simulink model "M10B39"  (R2016b)
settings: Solver=ode23tb  StartTime=0.0  StopTime=20  FixedStep=0.001  MaxStep=0.01  RelTol=1e-3  EnableMultiTasking=on
InitFcn:
  | initAll
values from neighbouring files (symbols this model uses):
  SgridB = 100    [initAll.m]
  wB = 2*pi*fB    (= 314.159265359)    [initAll.m]
  YY_load = full(YY)    [powerflowcaculate.m]
undefined symbols (not defined in the file): Geninit
libraries: powerlib_meascontrol x10, simulink x1
(part 1 of 3)
settings Model: Creator=m  LastModifiedBy=LinSiQi
settings DataIOCC: LimitDataPoints=on  SaveFormat=Array  SignalLoggingSaveFormat=ModelDataLogs  SignalLoggingName=sigsOut
settings OptimizationCC: ExpressionDepthLimit=2147483647  LifeSpan=inf
settings DebuggingCC: SaveWithParameterizedLinksMsg=none  UnderspecifiedInitializationDetection=Classic  MergeDetectMultiDrivingBlocksExec=none  SignalResolutionControl=TryResolveAllWithWarning  MultiTaskDSMMsg=warning  MultiTaskCondExecSysMsg=none  FcnCallInpInsideContextMsg=warning  StateNameClashWarn=warning  SFUnexpectedBacktrackingDiag=warning  SFNoUnconditionalDefaultTransitionDiag=warning  SFExecutionAtInitializationDiag=none
settings HardwareCC: ProdBitPerPointer=32  ProdBitPerSizeT=32  ProdBitPerPtrDiffT=32  ProdLargestAtomicFloat=None  ProdIntDivRoundTo=Undefined  ProdEndianess=Unspecified  ProdWordSize=32  ProdHWDeviceType=32-bit Generic  TargetUnknown=on
settings ModelReferenceCC: PropagateSignalLabelsOutOfModel=off
settings GRTTargetCC: TargetLangStandard=C89/C90 (ANSI)  CombineOutputUpdateFcns=off  GRTInterface=on
settings ConfigComp: CovMetricSettings=dw  CovSaveCumulativeToWorkspaceVar=on  CovSaveSingleToWorkspaceVar=on  CovExternalEMLEnable=off  CovSFcnEnable=off

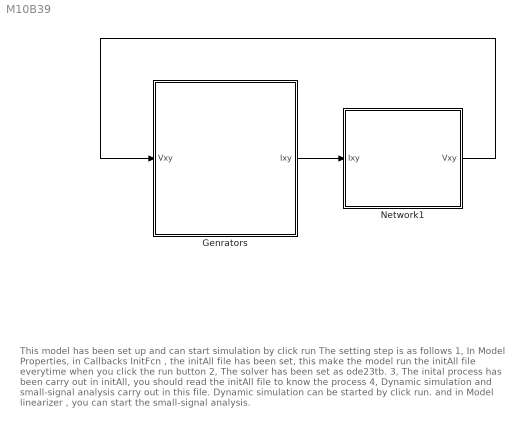
== system M10B39 ==
  note: This model has been set up and can start simulation by click run
      |
      | The setting step is as follows
      | 1, In Model Properties, in Callbacks InitFcn , the initAll file has been set, this make the model run the initAll file everytime when you click the run button
      |
      | 2, The solver has been set as ode23tb.
      |
      | 3, The inital process has been carry out in initAll, you should read the initAll file to know the process
      |
      | 4, Dynamic simulation and small-signal analysis carry out in this file. Dynamic simulation can be started by click run. and in Model linearizer , you can start the small-signal analysis.
  Genrators : Subsystem
  Network1 : Subsystem  mask{YY_load=YY_load, ng=10}
  wires:
  Genrators/1(Ixy) -> Network1/1(Ixy)
  Network1/1(Vxy) -> Genrators/1(Vxy)

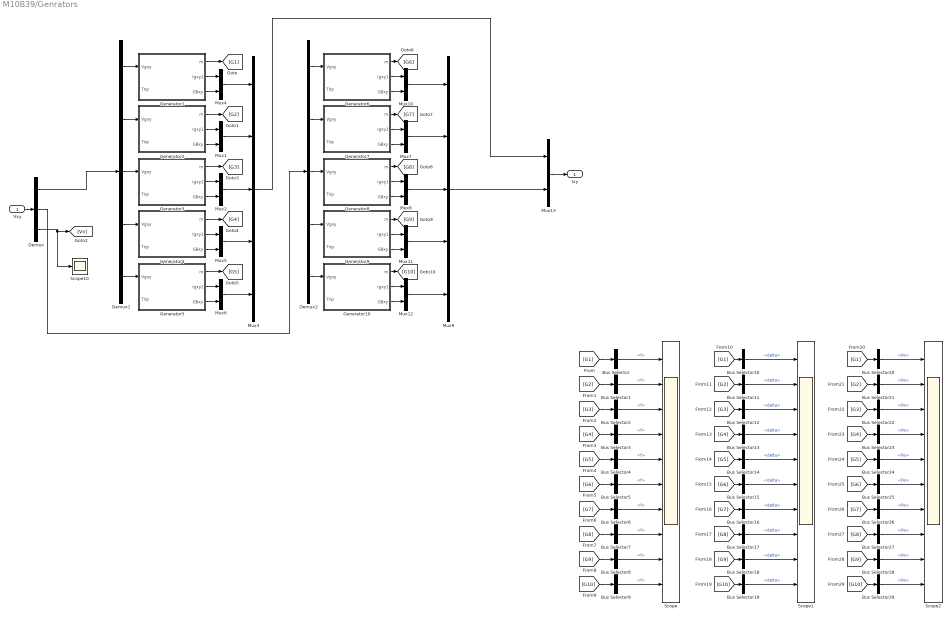
== system M10B39/Genrators ==
  Vxy : Inport
  Bus Selector{,1..9} (10 alike) : BusSelector  OutputSignals=f
  Bus Selector{10..19} (10 alike) : BusSelector  OutputSignals=delta
  Bus Selector{20..29} (10 alike) : BusSelector  OutputSignals=Pe
  Demux : Demux  Outputs=[10 10 29]
      settings: DisplayOption=none
  Demux1 : Demux  Outputs=5
      settings: DisplayOption=none
  Demux2 : Demux  Outputs=5
      settings: DisplayOption=none
  Generator1 : Subsystem  mask{wB=wB, SgenB=Geninit.SgenB(1), SgridB=SgridB, Xq=Geninit.Xq(1), Xq1=Geninit.Xq1(1), Xq11=Geninit.Xq11(1), Tq0=Geninit.Tq0(1), Tq10=Geninit.Tq10(1), Eq10=Geninit.Eq1(1), Eq110=Geninit.Eq11(1), Xd=Geninit.Xd(1), Xd1=Geninit.Xd1(1), Xd11=Geninit.Xd11(1), Td0=Geninit.Td0(1), Td10=Geninit.Td10(1), Ed10=Geninit.Ed1(1), Ed110=Geninit.Ed11(1), H=Geninit.Tj(1), D=Geninit.D(1), delta0=Geninit.Delta(1), w0=1, Pm0=Geninit.Pm0(1), Ka=Geninit.Ka(1), Tb=Geninit.Tb(1), Tc=Geninit.Tc(1), Efmax=Geninit.Efmax(1), Efmin=Geninit.Efmin(1), Vref=Geninit.Vref(1), Ef10=Geninit.Vf1(1), S_PSS=Geninit.EnablePSS(1), Kpss=Geninit.kpss(1), Tw_P=Geninit.Tw_P(1), T1_P=Geninit.T1_P(1), T2_P=Geninit.T2_P(1), T3_P=Geninit.T3_P(1), T4_P=Geninit.T4_P(1), Upmax=Geninit.Upmax(1), Upmin=Geninit.Upmin(1), S_Gov=Geninit.Enablegov(1), a_G=Geninit.a_G(1), b_G=Geninit.b_G(1), Tg_G=Geninit.Tg_G(1), dPmax=Geninit.dPmax(1), dPmin=Geninit.dPmin(1)}
      mask prompts: S_PSS "Enable PSS"; Tw_P "Tw"; T1_P "T1"; T2_P "T2"; T3_P "T3"; T4_P "T4"; S_Gov "Enable Governor"; a_G "a"; b_G "b"; Tg_G "Tg"
      mask help: This is a six-order synchronous generator with exciter system, governor and PSS.
  Generator10 : Subsystem  mask{wB=wB, SgenB=Geninit.SgenB(10), SgridB=SgridB, Xq=Geninit.Xq(10), Xq1=Geninit.Xq1(10), Xq11=Geninit.Xq11(10), Tq0=Geninit.Tq0(10), Tq10=Geninit.Tq10(10), Eq10=Geninit.Eq1(10), Eq110=Geninit.Eq11(10), Xd=Geninit.Xd(10), Xd1=Geninit.Xd1(10), Xd11=Geninit.Xd11(10), Td0=Geninit.Td0(10), Td10=Geninit.Td10(10), Ed10=Geninit.Ed1(10), Ed110=Geninit.Ed11(10), H=Geninit.Tj(10), D=Geninit.D(10), delta0=Geninit.Delta(10), w0=1, Pm0=Geninit.Pm0(10), Ka=Geninit.Ka(10), Tb=Geninit.Tb(10), Tc=Geninit.Tc(10), Efmax=Geninit.Efmax(10), Efmin=Geninit.Efmin(10), Vref=Geninit.Vref(10), Ef10=Geninit.Vf1(10), S_PSS=Geninit.EnablePSS(10), Kpss=Geninit.kpss(10), Tw_P=Geninit.Tw_P(10), T1_P=Geninit.T1_P(10), T2_P=Geninit.T2_P(10), T3_P=Geninit.T3_P(10), T4_P=Geninit.T4_P(10), Upmax=Geninit.Upmax(10), Upmin=Geninit.Upmin(10), S_Gov=Geninit.Enablegov(10), a_G=Geninit.a_G(10), b_G=Geninit.b_G(10), Tg_G=Geninit.Tg_G(10), dPmax=Geninit.dPmax(10), dPmin=Geninit.dPmin(10)}
      mask prompts: S_PSS "Enable PSS"; Tw_P "Tw"; T1_P "T1"; T2_P "T2"; T3_P "T3"; T4_P "T4"; S_Gov "Enable Governor"; a_G "a"; b_G "b"; Tg_G "Tg"
      mask help: This is a six-order synchronous generator with exciter system, governor and PSS.
  Generator2 : Subsystem  mask{wB=wB, SgenB=Geninit.SgenB(2), SgridB=SgridB, Xq=Geninit.Xq(2), Xq1=Geninit.Xq1(2), Xq11=Geninit.Xq11(2), Tq0=Geninit.Tq0(2), Tq10=Geninit.Tq10(2), Eq10=Geninit.Eq1(2), Eq110=Geninit.Eq11(2), Xd=Geninit.Xd(2), Xd1=Geninit.Xd1(2), Xd11=Geninit.Xd11(2), Td0=Geninit.Td0(2), Td10=Geninit.Td10(2), Ed10=Geninit.Ed1(2), Ed110=Geninit.Ed11(2), H=Geninit.Tj(2), D=Geninit.D(2), delta0=Geninit.Delta(2), w0=1, Pm0=Geninit.Pm0(2), Ka=Geninit.Ka(2), Tb=Geninit.Tb(2), Tc=Geninit.Tc(2), Efmax=Geninit.Efmax(2), Efmin=Geninit.Efmin(2), Vref=Geninit.Vref(2), Ef10=Geninit.Vf1(2), S_PSS=Geninit.EnablePSS(2), Kpss=Geninit.kpss(2), Tw_P=Geninit.Tw_P(2), T1_P=Geninit.T1_P(2), T2_P=Geninit.T2_P(2), T3_P=Geninit.T3_P(2), T4_P=Geninit.T4_P(2), Upmax=Geninit.Upmax(2), Upmin=Geninit.Upmin(2), S_Gov=Geninit.Enablegov(2), a_G=Geninit.a_G(2), b_G=Geninit.b_G(2), Tg_G=Geninit.Tg_G(2), dPmax=Geninit.dPmax(2), dPmin=Geninit.dPmin(2)}
      mask prompts: S_PSS "Enable PSS"; Tw_P "Tw"; T1_P "T1"; T2_P "T2"; T3_P "T3"; T4_P "T4"; S_Gov "Enable Governor"; a_G "a"; b_G "b"; Tg_G "Tg"
      mask help: This is a six-order synchronous generator with exciter system, governor and PSS.
  Generator3 : Subsystem  mask{wB=wB, SgenB=Geninit.SgenB(3), SgridB=SgridB, Xq=Geninit.Xq(3), Xq1=Geninit.Xq1(3), Xq11=Geninit.Xq11(3), Tq0=Geninit.Tq0(3), Tq10=Geninit.Tq10(3), Eq10=Geninit.Eq1(3), Eq110=Geninit.Eq11(3), Xd=Geninit.Xd(3), Xd1=Geninit.Xd1(3), Xd11=Geninit.Xd11(3), Td0=Geninit.Td0(3), Td10=Geninit.Td10(3), Ed10=Geninit.Ed1(3), Ed110=Geninit.Ed11(3), H=Geninit.Tj(3), D=Geninit.D(3), delta0=Geninit.Delta(3), w0=1, Pm0=Geninit.Pm0(3), Ka=Geninit.Ka(3), Tb=Geninit.Tb(3), Tc=Geninit.Tc(3), Efmax=Geninit.Efmax(3), Efmin=Geninit.Efmin(3), Vref=Geninit.Vref(3), Ef10=Geninit.Vf1(3), S_PSS=Geninit.EnablePSS(3), Kpss=Geninit.kpss(3), Tw_P=Geninit.Tw_P(3), T1_P=Geninit.T1_P(3), T2_P=Geninit.T2_P(3), T3_P=Geninit.T3_P(3), T4_P=Geninit.T4_P(3), Upmax=Geninit.Upmax(3), Upmin=Geninit.Upmin(3), S_Gov=Geninit.Enablegov(3), a_G=Geninit.a_G(3), b_G=Geninit.b_G(3), Tg_G=Geninit.Tg_G(3), dPmax=Geninit.dPmax(3), dPmin=Geninit.dPmin(3)}
      mask prompts: S_PSS "Enable PSS"; Tw_P "Tw"; T1_P "T1"; T2_P "T2"; T3_P "T3"; T4_P "T4"; S_Gov "Enable Governor"; a_G "a"; b_G "b"; Tg_G "Tg"
      mask help: This is a six-order synchronous generator with exciter system, governor and PSS.
  Generator4 : Subsystem  mask{wB=wB, SgenB=Geninit.SgenB(4), SgridB=SgridB, Xq=Geninit.Xq(4), Xq1=Geninit.Xq1(4), Xq11=Geninit.Xq11(4), Tq0=Geninit.Tq0(4), Tq10=Geninit.Tq10(4), Eq10=Geninit.Eq1(4), Eq110=Geninit.Eq11(4), Xd=Geninit.Xd(4), Xd1=Geninit.Xd1(4), Xd11=Geninit.Xd11(4), Td0=Geninit.Td0(4), Td10=Geninit.Td10(4), Ed10=Geninit.Ed1(4), Ed110=Geninit.Ed11(4), H=Geninit.Tj(4), D=Geninit.D(4), delta0=Geninit.Delta(4), w0=1, Pm0=Geninit.Pm0(4), Ka=Geninit.Ka(4), Tb=Geninit.Tb(4), Tc=Geninit.Tc(4), Efmax=Geninit.Efmax(4), Efmin=Geninit.Efmin(4), Vref=Geninit.Vref(4), Ef10=Geninit.Vf1(4), S_PSS=Geninit.EnablePSS(4), Kpss=Geninit.kpss(4), Tw_P=Geninit.Tw_P(4), T1_P=Geninit.T1_P(4), T2_P=Geninit.T2_P(4), T3_P=Geninit.T3_P(4), T4_P=Geninit.T4_P(4), Upmax=Geninit.Upmax(4), Upmin=Geninit.Upmin(4), S_Gov=Geninit.Enablegov(4), a_G=Geninit.a_G(4), b_G=Geninit.b_G(4), Tg_G=Geninit.Tg_G(4), dPmax=Geninit.dPmax(4), dPmin=Geninit.dPmin(4)}
      mask prompts: S_PSS "Enable PSS"; Tw_P "Tw"; T1_P "T1"; T2_P "T2"; T3_P "T3"; T4_P "T4"; S_Gov "Enable Governor"; a_G "a"; b_G "b"; Tg_G "Tg"
      mask help: This is a six-order synchronous generator with exciter system, governor and PSS.
  Generator5 : Subsystem  mask{wB=wB, SgenB=Geninit.SgenB(5), SgridB=SgridB, Xq=Geninit.Xq(5), Xq1=Geninit.Xq1(5), Xq11=Geninit.Xq11(5), Tq0=Geninit.Tq0(5), Tq10=Geninit.Tq10(5), Eq10=Geninit.Eq1(5), Eq110=Geninit.Eq11(5), Xd=Geninit.Xd(5), Xd1=Geninit.Xd1(5), Xd11=Geninit.Xd11(5), Td0=Geninit.Td0(5), Td10=Geninit.Td10(5), Ed10=Geninit.Ed1(5), Ed110=Geninit.Ed11(5), H=Geninit.Tj(5), D=Geninit.D(5), delta0=Geninit.Delta(5), w0=1, Pm0=Geninit.Pm0(5), Ka=Geninit.Ka(5), Tb=Geninit.Tb(5), Tc=Geninit.Tc(5), Efmax=Geninit.Efmax(5), Efmin=Geninit.Efmin(5), Vref=Geninit.Vref(5), Ef10=Geninit.Vf1(5), S_PSS=Geninit.EnablePSS(5), Kpss=Geninit.kpss(5), Tw_P=Geninit.Tw_P(5), T1_P=Geninit.T1_P(5), T2_P=Geninit.T2_P(5), T3_P=Geninit.T3_P(5), T4_P=Geninit.T4_P(5), Upmax=Geninit.Upmax(5), Upmin=Geninit.Upmin(5), S_Gov=Geninit.Enablegov(5), a_G=Geninit.a_G(5), b_G=Geninit.b_G(5), Tg_G=Geninit.Tg_G(5), dPmax=Geninit.dPmax(5), dPmin=Geninit.dPmin(5)}
      mask prompts: S_PSS "Enable PSS"; Tw_P "Tw"; T1_P "T1"; T2_P "T2"; T3_P "T3"; T4_P "T4"; S_Gov "Enable Governor"; a_G "a"; b_G "b"; Tg_G "Tg"
      mask help: This is a six-order synchronous generator with exciter system, governor and PSS.
  Generator6 : Subsystem  mask{wB=wB, SgenB=Geninit.SgenB(6), SgridB=SgridB, Xq=Geninit.Xq(6), Xq1=Geninit.Xq1(6), Xq11=Geninit.Xq11(6), Tq0=Geninit.Tq0(6), Tq10=Geninit.Tq10(6), Eq10=Geninit.Eq1(6), Eq110=Geninit.Eq11(6), Xd=Geninit.Xd(6), Xd1=Geninit.Xd1(6), Xd11=Geninit.Xd11(6), Td0=Geninit.Td0(6), Td10=Geninit.Td10(6), Ed10=Geninit.Ed1(6), Ed110=Geninit.Ed11(6), H=Geninit.Tj(6), D=Geninit.D(6), delta0=Geninit.Delta(6), w0=1, Pm0=Geninit.Pm0(6), Ka=Geninit.Ka(6), Tb=Geninit.Tb(6), Tc=Geninit.Tc(6), Efmax=Geninit.Efmax(6), Efmin=Geninit.Efmin(6), Vref=Geninit.Vref(6), Ef10=Geninit.Vf1(6), S_PSS=Geninit.EnablePSS(6), Kpss=Geninit.kpss(6), Tw_P=Geninit.Tw_P(6), T1_P=Geninit.T1_P(6), T2_P=Geninit.T2_P(6), T3_P=Geninit.T3_P(6), T4_P=Geninit.T4_P(6), Upmax=Geninit.Upmax(6), Upmin=Geninit.Upmin(6), S_Gov=Geninit.Enablegov(6), a_G=Geninit.a_G(6), b_G=Geninit.b_G(6), Tg_G=Geninit.Tg_G(6), dPmax=Geninit.dPmax(6), dPmin=Geninit.dPmin(6)}
      mask prompts: S_PSS "Enable PSS"; Tw_P "Tw"; T1_P "T1"; T2_P "T2"; T3_P "T3"; T4_P "T4"; S_Gov "Enable Governor"; a_G "a"; b_G "b"; Tg_G "Tg"
      mask help: This is a six-order synchronous generator with exciter system, governor and PSS.
  Generator7 : Subsystem  mask{wB=wB, SgenB=Geninit.SgenB(7), SgridB=SgridB, Xq=Geninit.Xq(7), Xq1=Geninit.Xq1(7), Xq11=Geninit.Xq11(7), Tq0=Geninit.Tq0(7), Tq10=Geninit.Tq10(7), Eq10=Geninit.Eq1(7), Eq110=Geninit.Eq11(7), Xd=Geninit.Xd(7), Xd1=Geninit.Xd1(7), Xd11=Geninit.Xd11(7), Td0=Geninit.Td0(7), Td10=Geninit.Td10(7), Ed10=Geninit.Ed1(7), Ed110=Geninit.Ed11(7), H=Geninit.Tj(7), D=Geninit.D(7), delta0=Geninit.Delta(7), w0=1, Pm0=Geninit.Pm0(7), Ka=Geninit.Ka(7), Tb=Geninit.Tb(7), Tc=Geninit.Tc(7), Efmax=Geninit.Efmax(7), Efmin=Geninit.Efmin(7), Vref=Geninit.Vref(7), Ef10=Geninit.Vf1(7), S_PSS=Geninit.EnablePSS(7), Kpss=Geninit.kpss(7), Tw_P=Geninit.Tw_P(7), T1_P=Geninit.T1_P(7), T2_P=Geninit.T2_P(7), T3_P=Geninit.T3_P(7), T4_P=Geninit.T4_P(7), Upmax=Geninit.Upmax(7), Upmin=Geninit.Upmin(7), S_Gov=Geninit.Enablegov(7), a_G=Geninit.a_G(7), b_G=Geninit.b_G(7), Tg_G=Geninit.Tg_G(7), dPmax=Geninit.dPmax(7), dPmin=Geninit.dPmin(7)}
      mask prompts: S_PSS "Enable PSS"; Tw_P "Tw"; T1_P "T1"; T2_P "T2"; T3_P "T3"; T4_P "T4"; S_Gov "Enable Governor"; a_G "a"; b_G "b"; Tg_G "Tg"
      mask help: This is a six-order synchronous generator with exciter system, governor and PSS.
  Generator8 : Subsystem  mask{wB=wB, SgenB=Geninit.SgenB(8), SgridB=SgridB, Xq=Geninit.Xq(8), Xq1=Geninit.Xq1(8), Xq11=Geninit.Xq11(8), Tq0=Geninit.Tq0(8), Tq10=Geninit.Tq10(8), Eq10=Geninit.Eq1(8), Eq110=Geninit.Eq11(8), Xd=Geninit.Xd(8), Xd1=Geninit.Xd1(8), Xd11=Geninit.Xd11(8), Td0=Geninit.Td0(8), Td10=Geninit.Td10(8), Ed10=Geninit.Ed1(8), Ed110=Geninit.Ed11(8), H=Geninit.Tj(8), D=Geninit.D(8), delta0=Geninit.Delta(8), w0=1, Pm0=Geninit.Pm0(8), Ka=Geninit.Ka(8), Tb=Geninit.Tb(8), Tc=Geninit.Tc(8), Efmax=Geninit.Efmax(8), Efmin=Geninit.Efmin(8), Vref=Geninit.Vref(8), Ef10=Geninit.Vf1(8), S_PSS=Geninit.EnablePSS(8), Kpss=Geninit.kpss(8), Tw_P=Geninit.Tw_P(8), T1_P=Geninit.T1_P(8), T2_P=Geninit.T2_P(8), T3_P=Geninit.T3_P(8), T4_P=Geninit.T4_P(8), Upmax=Geninit.Upmax(8), Upmin=Geninit.Upmin(8), S_Gov=Geninit.Enablegov(8), a_G=Geninit.a_G(8), b_G=Geninit.b_G(8), Tg_G=Geninit.Tg_G(8), dPmax=Geninit.dPmax(8), dPmin=Geninit.dPmin(8)}
      mask prompts: S_PSS "Enable PSS"; Tw_P "Tw"; T1_P "T1"; T2_P "T2"; T3_P "T3"; T4_P "T4"; S_Gov "Enable Governor"; a_G "a"; b_G "b"; Tg_G "Tg"
      mask help: This is a six-order synchronous generator with exciter system, governor and PSS.
  Generator9 : Subsystem  mask{wB=wB, SgenB=Geninit.SgenB(9), SgridB=SgridB, Xq=Geninit.Xq(9), Xq1=Geninit.Xq1(9), Xq11=Geninit.Xq11(9), Tq0=Geninit.Tq0(9), Tq10=Geninit.Tq10(9), Eq10=Geninit.Eq1(9), Eq110=Geninit.Eq11(9), Xd=Geninit.Xd(9), Xd1=Geninit.Xd1(9), Xd11=Geninit.Xd11(9), Td0=Geninit.Td0(9), Td10=Geninit.Td10(9), Ed10=Geninit.Ed1(9), Ed110=Geninit.Ed11(9), H=Geninit.Tj(9), D=Geninit.D(9), delta0=Geninit.Delta(9), w0=1, Pm0=Geninit.Pm0(9), Ka=Geninit.Ka(9), Tb=Geninit.Tb(9), Tc=Geninit.Tc(9), Efmax=Geninit.Efmax(9), Efmin=Geninit.Efmin(9), Vref=Geninit.Vref(9), Ef10=Geninit.Vf1(9), S_PSS=Geninit.EnablePSS(9), Kpss=Geninit.kpss(9), Tw_P=Geninit.Tw_P(9), T1_P=Geninit.T1_P(9), T2_P=Geninit.T2_P(9), T3_P=Geninit.T3_P(9), T4_P=Geninit.T4_P(9), Upmax=Geninit.Upmax(9), Upmin=Geninit.Upmin(9), S_Gov=Geninit.Enablegov(9), a_G=Geninit.a_G(9), b_G=Geninit.b_G(9), Tg_G=Geninit.Tg_G(9), dPmax=Geninit.dPmax(9), dPmin=Geninit.dPmin(9)}
      mask prompts: S_PSS "Enable PSS"; Tw_P "Tw"; T1_P "T1"; T2_P "T2"; T3_P "T3"; T4_P "T4"; S_Gov "Enable Governor"; a_G "a"; b_G "b"; Tg_G "Tg"
      mask help: This is a six-order synchronous generator with exciter system, governor and PSS.
  Mux{1..2,4..8,10..13} (11 alike) : Mux  Inputs=2
  Mux3 : Mux  Inputs=5
  Mux9 : Mux  Inputs=5
  Scope : Scope  NumInputPorts=10
  Scope1 : Scope  NumInputPorts=10
  Scope10 : Scope
  Scope2 : Scope  NumInputPorts=10
  Ixy : Outport
  wires:
  Generator1/2(Igxy1) -> Mux4/1
  Generator1/3(GBxy) -> Mux4/2
  Generator3/2(Igxy1) -> Mux2/1
  Generator3/3(GBxy) -> Mux2/2
  Generator4/3(GBxy) -> Mux5/2
  Generator5/2(Igxy1) -> Mux6/1
  Generator5/3(GBxy) -> Mux6/2
  Mux4/1 -> Mux3/1
  Mux1/1 -> Mux3/2
  Mux2/1 -> Mux3/3
  Mux5/1 -> Mux3/4
  Mux6/1 -> Mux3/5
  Demux1/1 -> Generator1/1(Vgxy)
  Demux1/2 -> Generator2/1(Vgxy)
  Demux1/3 -> Generator3/1(Vgxy)
  Demux1/4 -> Generator4/1(Vgxy)
  Demux1/5 -> Generator5/1(Vgxy)
  Generator6/2(Igxy1) -> Mux10/1
  Generator6/3(GBxy) -> Mux10/2
  Generator7/2(Igxy1) -> Mux7/1
  Generator7/3(GBxy) -> Mux7/2
  Generator8/2(Igxy1) -> Mux8/1
  Generator8/3(GBxy) -> Mux8/2
  Generator9/2(Igxy1) -> Mux11/1
  Generator9/3(GBxy) -> Mux11/2
  Generator10/2(Igxy1) -> Mux12/1
  Generator10/3(GBxy) -> Mux12/2
  Mux10/1 -> Mux9/1
  Mux7/1 -> Mux9/2
  Mux8/1 -> Mux9/3
  Mux11/1 -> Mux9/4
  Mux12/1 -> Mux9/5
  Demux2/1 -> Generator6/1(Vgxy)
  Demux2/2 -> Generator7/1(Vgxy)
  Demux2/3 -> Generator8/1(Vgxy)
  Demux2/4 -> Generator9/1(Vgxy)
  Demux2/5 -> Generator10/1(Vgxy)
  Mux13/1 -> Ixy/1
  Mux9/1 -> Mux13/2
  Mux3/1 -> Mux13/1
  Vxy/1 -> Demux/1
  Demux/1 -> Demux1/1
  Demux/2 -> Demux2/1
  Demux/3 -> [Vn], Scope10/1
  Generator2/2(Igxy1) -> Mux1/1
  Generator2/3(GBxy) -> Mux1/2
  Generator4/2(Igxy1) -> Mux5/1
  Generator1/1(m) -> [G1]
  Generator2/1(m) -> [G2]
  Generator3/1(m) -> [G3]
  Generator4/1(m) -> [G4]
  Generator5/1(m) -> [G5]
  Generator6/1(m) -> [G6]
  Generator7/1(m) -> [G7]
  Generator8/1(m) -> [G8]
  Generator9/1(m) -> [G9]
  Generator10/1(m) -> [G10]
  [G1] -> Bus Selector/1
  [G2] -> Bus Selector1/1
  [G3] -> Bus Selector2/1
  [G4] -> Bus Selector3/1
  [G5] -> Bus Selector4/1
  [G6] -> Bus Selector5/1
  [G7] -> Bus Selector6/1
  [G8] -> Bus Selector7/1
  [G9] -> Bus Selector8/1
  [G10] -> Bus Selector9/1
  Bus Selector/1 -> Scope/1  "<f>"
  Bus Selector1/1 -> Scope/2  "<f>"
  Bus Selector2/1 -> Scope/3  "<f>"
  Bus Selector3/1 -> Scope/4  "<f>"
  Bus Selector4/1 -> Scope/5  "<f>"
  Bus Selector5/1 -> Scope/6  "<f>"
  Bus Selector6/1 -> Scope/7  "<f>"
  Bus Selector7/1 -> Scope/8  "<f>"
  Bus Selector8/1 -> Scope/9  "<f>"
  Bus Selector9/1 -> Scope/10  "<f>"
  [G1] -> Bus Selector10/1
  [G2] -> Bus Selector11/1
  [G3] -> Bus Selector12/1
  [G4] -> Bus Selector13/1
  [G5] -> Bus Selector14/1
  [G6] -> Bus Selector15/1
  [G7] -> Bus Selector16/1
  [G8] -> Bus Selector17/1
  [G9] -> Bus Selector18/1
  [G10] -> Bus Selector19/1
  Bus Selector19/1 -> Scope1/10  "<delta>"
  Bus Selector18/1 -> Scope1/9  "<delta>"
  Bus Selector17/1 -> Scope1/8  "<delta>"
  Bus Selector16/1 -> Scope1/7  "<delta>"
  Bus Selector15/1 -> Scope1/6  "<delta>"
  Bus Selector14/1 -> Scope1/5  "<delta>"
  Bus Selector13/1 -> Scope1/4  "<delta>"
  Bus Selector12/1 -> Scope1/3  "<delta>"
  Bus Selector11/1 -> Scope1/2  "<delta>"
  Bus Selector10/1 -> Scope1/1  "<delta>"
  [G8] -> Bus Selector27/1
  [G1] -> Bus Selector20/1
  [G2] -> Bus Selector21/1
  [G7] -> Bus Selector26/1
  [G10] -> Bus Selector29/1
  [G9] -> Bus Selector28/1
  [G4] -> Bus Selector23/1
  [G3] -> Bus Selector22/1
  [G6] -> Bus Selector25/1
  [G5] -> Bus Selector24/1
  Bus Selector20/1 -> Scope2/1  "<Pe>"
  Bus Selector21/1 -> Scope2/2  "<Pe>"
  Bus Selector22/1 -> Scope2/3  "<Pe>"
  Bus Selector23/1 -> Scope2/4  "<Pe>"
  Bus Selector24/1 -> Scope2/5  "<Pe>"
  Bus Selector25/1 -> Scope2/6  "<Pe>"
  Bus Selector26/1 -> Scope2/7  "<Pe>"
  Bus Selector27/1 -> Scope2/8  "<Pe>"
  Bus Selector28/1 -> Scope2/9  "<Pe>"
  Bus Selector29/1 -> Scope2/10  "<Pe>"

== system M10B39/Network1 ==
  Ixy : Inport
  Clock : Clock
  Mux : Mux  Inputs=2
  S-Function : S-Function  FunctionName=TS_net_1_new  Parameters=YY_load,ng  SFunctionDeploymentMode=off  EnableBusSupport=off
  S-Function Examples : simulink/User-Defined Functions/S-Function Examples  Commented=on
  S-Function1 : S-Function  Commented=on  Parameters=YY_load,ng  SFunctionDeploymentMode=off  EnableBusSupport=off
  Vxy : Outport
  wires:
  Clock/1 -> Mux/1
  Ixy/1 -> Mux/2
  Mux/1 -> S-Function/1
  S-Function/1 -> Vxy/1

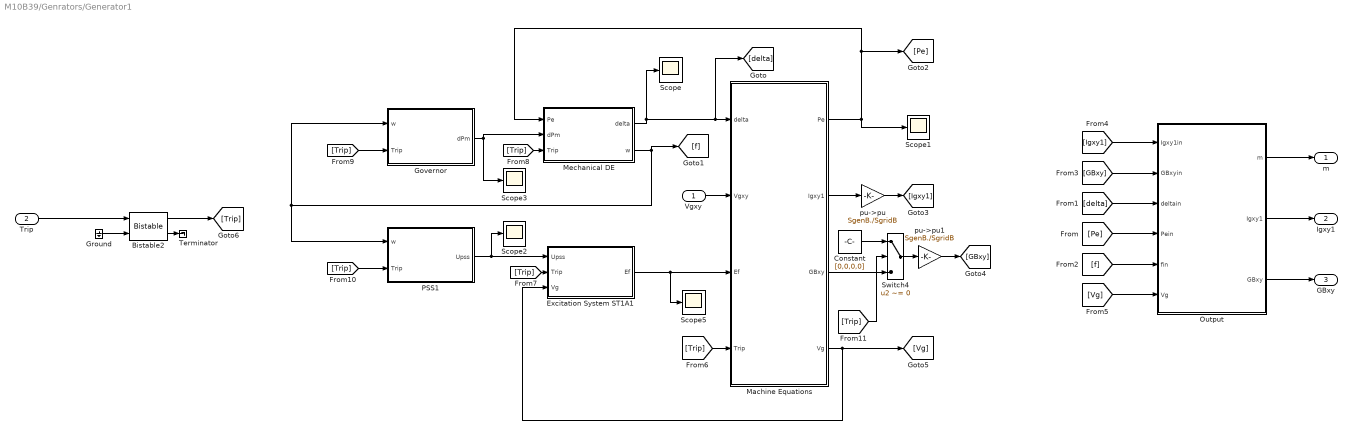
== system M10B39/Genrators/Generator1 ==
  Vgxy : Inport
  Trip : Inport  Port=2
  Bistable2 : powerlib_meascontrol/Logic/Bistable  Qpriority=Set  ic=0  Ts=0
  Constant : Constant  Value=[0,0,0,0]
  Excitation System ST1A1 : Subsystem
  Governor : Subsystem
  Ground : Ground
  "Machine Equations " : Subsystem
  Mechanical DE : Subsystem
  Output : Subsystem
  PSS1 : Subsystem
  Scope{,1..3,5} (5 alike) : Scope
  Switch4 : Switch  Criteria=u2 ~= 0  Threshold=0.5  SaturateOnIntegerOverflow=on
  Terminator : Terminator
  pu->pu : Gain  Gain=SgenB./SgridB
  pu->pu1 : Gain  Gain=SgenB./SgridB
  m : Outport
  Igxy1 : Outport  Port=2
  GBxy : Outport  Port=3
  wires:
  pu->pu1/1 -> [GBxy]
  pu->pu/1 -> [Igxy1]
  "Machine Equations "/3(GBxy) -> Switch4/3
  Constant/1 -> Switch4/1
  Switch4/1 -> pu->pu1/1
  [Trip] -> Switch4/2
  [Trip] -> PSS1/2(Trip)
  [Trip] -> Governor/2(Trip)
  [Trip] -> Mechanical DE/3(Trip)
  [Trip] -> Excitation System ST1A1/2(Trip)
  [Trip] -> "Machine Equations "/4(Trip)
  Bistable2/2 -> Terminator/1
  Trip/1 -> Bistable2/1
  Ground/1 -> Bistable2/2
  Bistable2/1 -> [Trip]
  [Vg] -> Output/6(Vg)
  Output/1(m) -> m/1
  Output/3(GBxy) -> GBxy/1
  Output/2(Igxy1) -> Igxy1/1
  [Igxy1] -> Output/1(Igxy1in)
  [GBxy] -> Output/2(GBxyin)
  [delta] -> Output/3(deltain)
  [f] -> Output/5(fin)
  [Pe] -> Output/4(Pein)
  Mechanical DE/1(delta) -> "Machine Equations "/1(delta), [delta], Scope/1
  Governor/1(dPm) -> Scope3/1, Mechanical DE/2(dPm)
  PSS1/1(Upss) -> Scope2/1, Excitation System ST1A1/1(Upss)
  Mechanical DE/2(w) -> [f], PSS1/1(w), Governor/1(w)
  "Machine Equations "/2(Igxy1) -> pu->pu/1
  Vgxy/1 -> "Machine Equations "/2(Vgxy)
  "Machine Equations "/4(Vg) -> [Vg], Excitation System ST1A1/3(Vg)
  "Machine Equations "/1(Pe) -> [Pe], Mechanical DE/1(Pe), Scope1/1
  Excitation System ST1A1/1(Ef) -> "Machine Equations "/3(Ef), Scope5/1

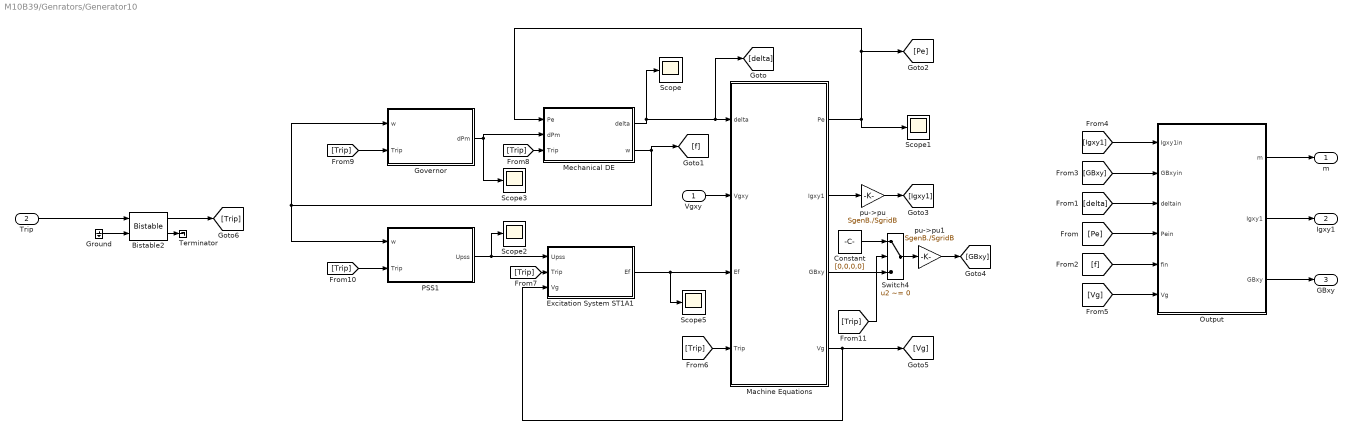
== system M10B39/Genrators/Generator10 ==
  Vgxy : Inport
  Trip : Inport  Port=2
  Bistable2 : powerlib_meascontrol/Logic/Bistable  Qpriority=Set  ic=0  Ts=0
  Constant : Constant  Value=[0,0,0,0]
  Excitation System ST1A1 : Subsystem
  Governor : Subsystem
  Ground : Ground
  "Machine Equations " : Subsystem
  Mechanical DE : Subsystem
  Output : Subsystem
  PSS1 : Subsystem
  Scope{,1..3,5} (5 alike) : Scope
  Switch4 : Switch  Criteria=u2 ~= 0  Threshold=0.5  SaturateOnIntegerOverflow=on
  Terminator : Terminator
  pu->pu : Gain  Gain=SgenB./SgridB
  pu->pu1 : Gain  Gain=SgenB./SgridB
  m : Outport
  Igxy1 : Outport  Port=2
  GBxy : Outport  Port=3
  wires:
  pu->pu1/1 -> [GBxy]
  pu->pu/1 -> [Igxy1]
  "Machine Equations "/3(GBxy) -> Switch4/3
  Constant/1 -> Switch4/1
  Switch4/1 -> pu->pu1/1
  [Trip] -> Switch4/2
  [Trip] -> PSS1/2(Trip)
  [Trip] -> Governor/2(Trip)
  [Trip] -> Mechanical DE/3(Trip)
  [Trip] -> Excitation System ST1A1/2(Trip)
  [Trip] -> "Machine Equations "/4(Trip)
  Bistable2/2 -> Terminator/1
  Trip/1 -> Bistable2/1
  Ground/1 -> Bistable2/2
  Bistable2/1 -> [Trip]
  [Vg] -> Output/6(Vg)
  Output/1(m) -> m/1
  Output/3(GBxy) -> GBxy/1
  Output/2(Igxy1) -> Igxy1/1
  [Igxy1] -> Output/1(Igxy1in)
  [GBxy] -> Output/2(GBxyin)
  [delta] -> Output/3(deltain)
  [f] -> Output/5(fin)
  [Pe] -> Output/4(Pein)
  Mechanical DE/1(delta) -> "Machine Equations "/1(delta), [delta], Scope/1
  Governor/1(dPm) -> Scope3/1, Mechanical DE/2(dPm)
  PSS1/1(Upss) -> Scope2/1, Excitation System ST1A1/1(Upss)
  Mechanical DE/2(w) -> [f], PSS1/1(w), Governor/1(w)
  "Machine Equations "/2(Igxy1) -> pu->pu/1
  Vgxy/1 -> "Machine Equations "/2(Vgxy)
  "Machine Equations "/4(Vg) -> [Vg], Excitation System ST1A1/3(Vg)
  "Machine Equations "/1(Pe) -> [Pe], Mechanical DE/1(Pe), Scope1/1
  Excitation System ST1A1/1(Ef) -> "Machine Equations "/3(Ef), Scope5/1

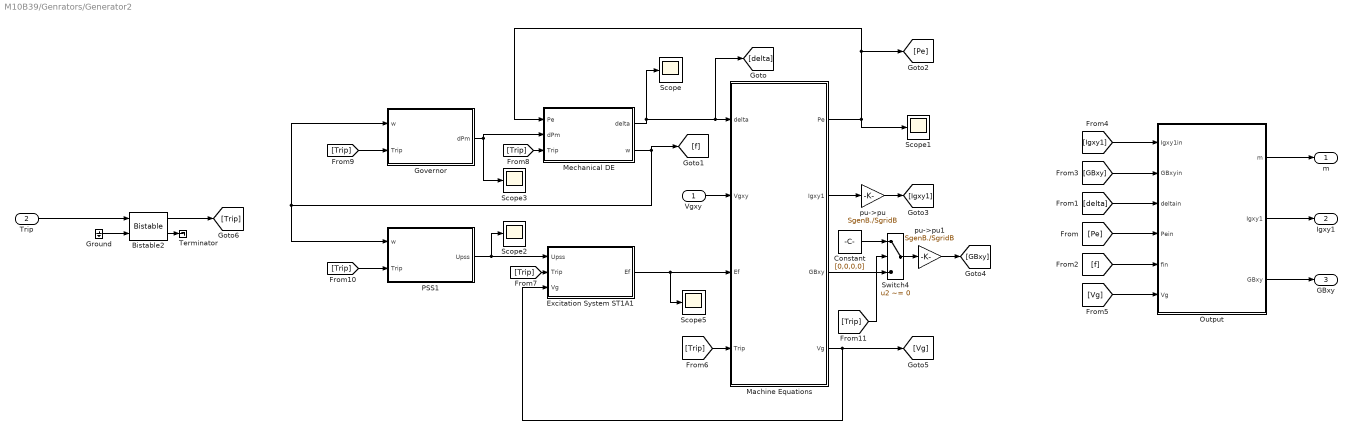
== system M10B39/Genrators/Generator2 ==
  Vgxy : Inport
  Trip : Inport  Port=2
  Bistable2 : powerlib_meascontrol/Logic/Bistable  Qpriority=Set  ic=0  Ts=0
  Constant : Constant  Value=[0,0,0,0]
  Excitation System ST1A1 : Subsystem
  Governor : Subsystem
  Ground : Ground
  "Machine Equations " : Subsystem
  Mechanical DE : Subsystem
  Output : Subsystem
  PSS1 : Subsystem
  Scope{,1..3,5} (5 alike) : Scope
  Switch4 : Switch  Criteria=u2 ~= 0  Threshold=0.5  SaturateOnIntegerOverflow=on
  Terminator : Terminator
  pu->pu : Gain  Gain=SgenB./SgridB
  pu->pu1 : Gain  Gain=SgenB./SgridB
  m : Outport
  Igxy1 : Outport  Port=2
  GBxy : Outport  Port=3
  wires:
  pu->pu1/1 -> [GBxy]
  pu->pu/1 -> [Igxy1]
  "Machine Equations "/3(GBxy) -> Switch4/3
  Constant/1 -> Switch4/1
  Switch4/1 -> pu->pu1/1
  [Trip] -> Switch4/2
  [Trip] -> PSS1/2(Trip)
  [Trip] -> Governor/2(Trip)
  [Trip] -> Mechanical DE/3(Trip)
  [Trip] -> Excitation System ST1A1/2(Trip)
  [Trip] -> "Machine Equations "/4(Trip)
  Bistable2/2 -> Terminator/1
  Trip/1 -> Bistable2/1
  Ground/1 -> Bistable2/2
  Bistable2/1 -> [Trip]
  [Vg] -> Output/6(Vg)
  Output/1(m) -> m/1
  Output/3(GBxy) -> GBxy/1
  Output/2(Igxy1) -> Igxy1/1
  [Igxy1] -> Output/1(Igxy1in)
  [GBxy] -> Output/2(GBxyin)
  [delta] -> Output/3(deltain)
  [f] -> Output/5(fin)
  [Pe] -> Output/4(Pein)
  Mechanical DE/1(delta) -> "Machine Equations "/1(delta), [delta], Scope/1
  Governor/1(dPm) -> Scope3/1, Mechanical DE/2(dPm)
  PSS1/1(Upss) -> Scope2/1, Excitation System ST1A1/1(Upss)
  Mechanical DE/2(w) -> [f], PSS1/1(w), Governor/1(w)
  "Machine Equations "/2(Igxy1) -> pu->pu/1
  Vgxy/1 -> "Machine Equations "/2(Vgxy)
  "Machine Equations "/4(Vg) -> [Vg], Excitation System ST1A1/3(Vg)
  "Machine Equations "/1(Pe) -> [Pe], Mechanical DE/1(Pe), Scope1/1
  Excitation System ST1A1/1(Ef) -> "Machine Equations "/3(Ef), Scope5/1

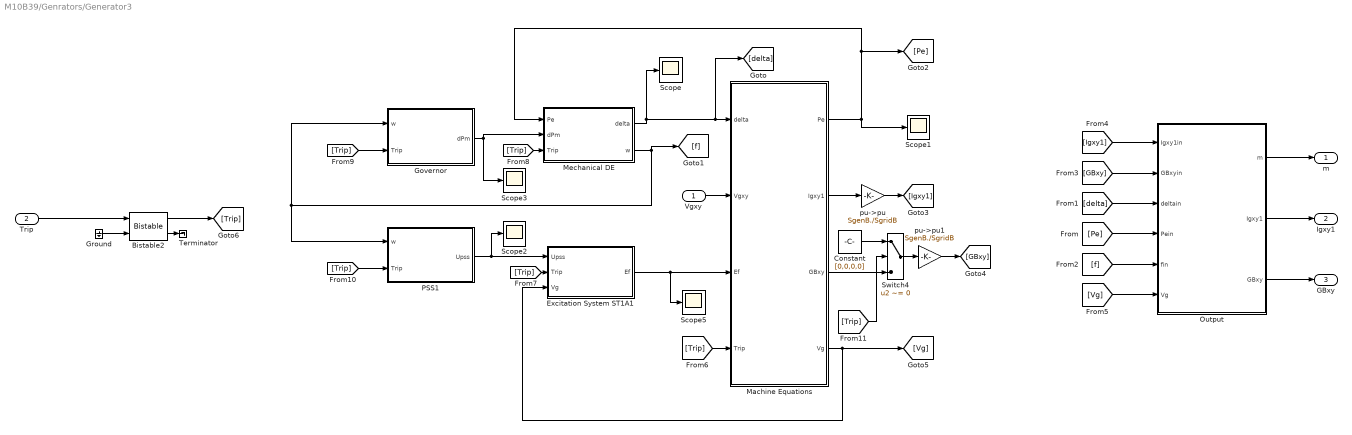
== system M10B39/Genrators/Generator3 ==
  Vgxy : Inport
  Trip : Inport  Port=2
  Bistable2 : powerlib_meascontrol/Logic/Bistable  Qpriority=Set  ic=0  Ts=0
  Constant : Constant  Value=[0,0,0,0]
  Excitation System ST1A1 : Subsystem
  Governor : Subsystem
  Ground : Ground
  "Machine Equations " : Subsystem
  Mechanical DE : Subsystem
  Output : Subsystem
  PSS1 : Subsystem
  Scope{,1..3,5} (5 alike) : Scope
  Switch4 : Switch  Criteria=u2 ~= 0  Threshold=0.5  SaturateOnIntegerOverflow=on
  Terminator : Terminator
  pu->pu : Gain  Gain=SgenB./SgridB
  pu->pu1 : Gain  Gain=SgenB./SgridB
  m : Outport
  Igxy1 : Outport  Port=2
  GBxy : Outport  Port=3
  wires:
  pu->pu1/1 -> [GBxy]
  pu->pu/1 -> [Igxy1]
  "Machine Equations "/3(GBxy) -> Switch4/3
  Constant/1 -> Switch4/1
  Switch4/1 -> pu->pu1/1
  [Trip] -> Switch4/2
  [Trip] -> PSS1/2(Trip)
  [Trip] -> Governor/2(Trip)
  [Trip] -> Mechanical DE/3(Trip)
  [Trip] -> Excitation System ST1A1/2(Trip)
  [Trip] -> "Machine Equations "/4(Trip)
  Bistable2/2 -> Terminator/1
  Trip/1 -> Bistable2/1
  Ground/1 -> Bistable2/2
  Bistable2/1 -> [Trip]
  [Vg] -> Output/6(Vg)
  Output/1(m) -> m/1
  Output/3(GBxy) -> GBxy/1
  Output/2(Igxy1) -> Igxy1/1
  [Igxy1] -> Output/1(Igxy1in)
  [GBxy] -> Output/2(GBxyin)
  [delta] -> Output/3(deltain)
  [f] -> Output/5(fin)
  [Pe] -> Output/4(Pein)
  Mechanical DE/1(delta) -> "Machine Equations "/1(delta), [delta], Scope/1
  Governor/1(dPm) -> Scope3/1, Mechanical DE/2(dPm)
  PSS1/1(Upss) -> Scope2/1, Excitation System ST1A1/1(Upss)
  Mechanical DE/2(w) -> [f], PSS1/1(w), Governor/1(w)
  "Machine Equations "/2(Igxy1) -> pu->pu/1
  Vgxy/1 -> "Machine Equations "/2(Vgxy)
  "Machine Equations "/4(Vg) -> [Vg], Excitation System ST1A1/3(Vg)
  "Machine Equations "/1(Pe) -> [Pe], Mechanical DE/1(Pe), Scope1/1
  Excitation System ST1A1/1(Ef) -> "Machine Equations "/3(Ef), Scope5/1

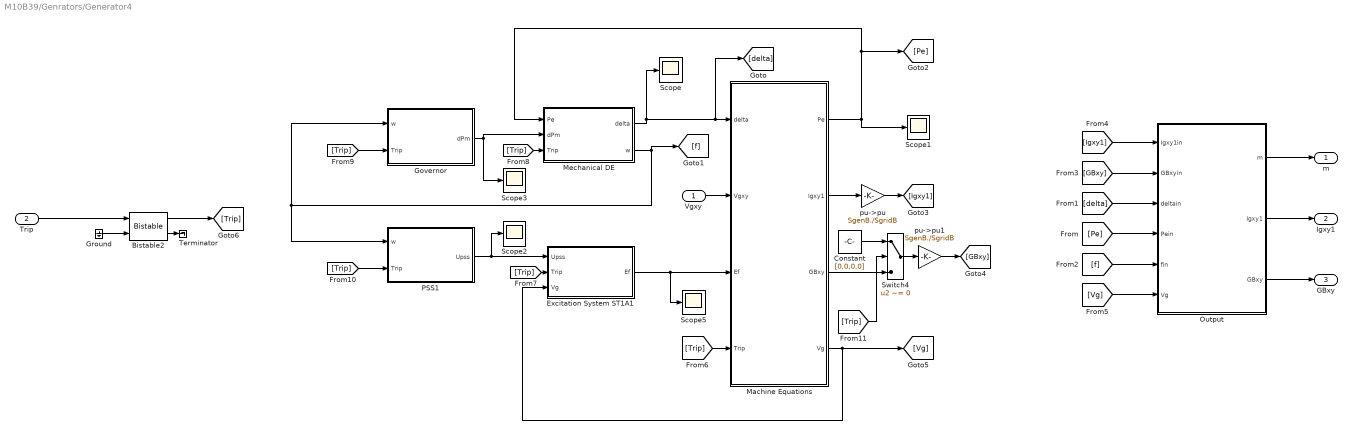
== system M10B39/Genrators/Generator4 ==
  Vgxy : Inport
  Trip : Inport  Port=2
  Bistable2 : powerlib_meascontrol/Logic/Bistable  Qpriority=Set  ic=0  Ts=0
  Constant : Constant  Value=[0,0,0,0]
  Excitation System ST1A1 : Subsystem
  Governor : Subsystem
  Ground : Ground
  "Machine Equations " : Subsystem
  Mechanical DE : Subsystem
  Output : Subsystem
  PSS1 : Subsystem
  Scope{,1..3,5} (5 alike) : Scope
  Switch4 : Switch  Criteria=u2 ~= 0  Threshold=0.5  SaturateOnIntegerOverflow=on
  Terminator : Terminator
  pu->pu : Gain  Gain=SgenB./SgridB
  pu->pu1 : Gain  Gain=SgenB./SgridB
  m : Outport
  Igxy1 : Outport  Port=2
  GBxy : Outport  Port=3
  wires:
  pu->pu1/1 -> [GBxy]
  pu->pu/1 -> [Igxy1]
  "Machine Equations "/3(GBxy) -> Switch4/3
  Constant/1 -> Switch4/1
  Switch4/1 -> pu->pu1/1
  [Trip] -> Switch4/2
  [Trip] -> PSS1/2(Trip)
  [Trip] -> Governor/2(Trip)
  [Trip] -> Mechanical DE/3(Trip)
  [Trip] -> Excitation System ST1A1/2(Trip)
  [Trip] -> "Machine Equations "/4(Trip)
  Bistable2/2 -> Terminator/1
  Trip/1 -> Bistable2/1
  Ground/1 -> Bistable2/2
  Bistable2/1 -> [Trip]
  [Vg] -> Output/6(Vg)
  Output/1(m) -> m/1
  Output/3(GBxy) -> GBxy/1
  Output/2(Igxy1) -> Igxy1/1
  [Igxy1] -> Output/1(Igxy1in)
  [GBxy] -> Output/2(GBxyin)
  [delta] -> Output/3(deltain)
  [f] -> Output/5(fin)
  [Pe] -> Output/4(Pein)
  Mechanical DE/1(delta) -> "Machine Equations "/1(delta), [delta], Scope/1
  Governor/1(dPm) -> Scope3/1, Mechanical DE/2(dPm)
  PSS1/1(Upss) -> Scope2/1, Excitation System ST1A1/1(Upss)
  Mechanical DE/2(w) -> [f], PSS1/1(w), Governor/1(w)
  "Machine Equations "/2(Igxy1) -> pu->pu/1
  Vgxy/1 -> "Machine Equations "/2(Vgxy)
  "Machine Equations "/4(Vg) -> [Vg], Excitation System ST1A1/3(Vg)
  "Machine Equations "/1(Pe) -> [Pe], Mechanical DE/1(Pe), Scope1/1
  Excitation System ST1A1/1(Ef) -> "Machine Equations "/3(Ef), Scope5/1

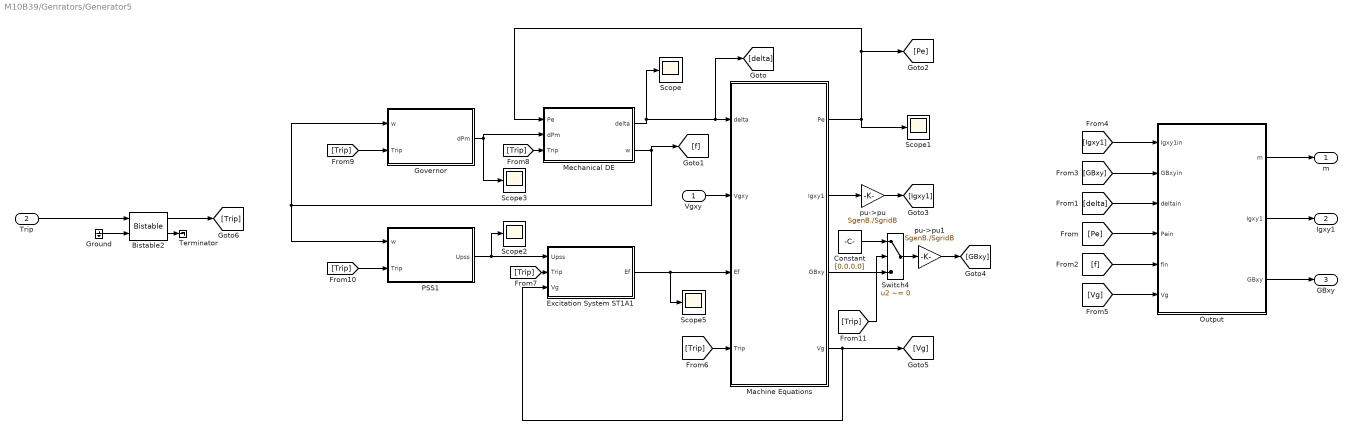
== system M10B39/Genrators/Generator5 ==
  Vgxy : Inport
  Trip : Inport  Port=2
  Bistable2 : powerlib_meascontrol/Logic/Bistable  Qpriority=Set  ic=0  Ts=0
  Constant : Constant  Value=[0,0,0,0]
  Excitation System ST1A1 : Subsystem
  Governor : Subsystem
  Ground : Ground
  "Machine Equations " : Subsystem
  Mechanical DE : Subsystem
  Output : Subsystem
  PSS1 : Subsystem
  Scope{,1..3,5} (5 alike) : Scope
  Switch4 : Switch  Criteria=u2 ~= 0  Threshold=0.5  SaturateOnIntegerOverflow=on
  Terminator : Terminator
  pu->pu : Gain  Gain=SgenB./SgridB
  pu->pu1 : Gain  Gain=SgenB./SgridB
  m : Outport
  Igxy1 : Outport  Port=2
  GBxy : Outport  Port=3
  wires:
  pu->pu1/1 -> [GBxy]
  pu->pu/1 -> [Igxy1]
  "Machine Equations "/3(GBxy) -> Switch4/3
  Constant/1 -> Switch4/1
  Switch4/1 -> pu->pu1/1
  [Trip] -> Switch4/2
  [Trip] -> PSS1/2(Trip)
  [Trip] -> Governor/2(Trip)
  [Trip] -> Mechanical DE/3(Trip)
  [Trip] -> Excitation System ST1A1/2(Trip)
  [Trip] -> "Machine Equations "/4(Trip)
  Bistable2/2 -> Terminator/1
  Trip/1 -> Bistable2/1
  Ground/1 -> Bistable2/2
  Bistable2/1 -> [Trip]
  [Vg] -> Output/6(Vg)
  Output/1(m) -> m/1
  Output/3(GBxy) -> GBxy/1
  Output/2(Igxy1) -> Igxy1/1
  [Igxy1] -> Output/1(Igxy1in)
  [GBxy] -> Output/2(GBxyin)
  [delta] -> Output/3(deltain)
  [f] -> Output/5(fin)
  [Pe] -> Output/4(Pein)
  Mechanical DE/1(delta) -> "Machine Equations "/1(delta), [delta], Scope/1
  Governor/1(dPm) -> Scope3/1, Mechanical DE/2(dPm)
  PSS1/1(Upss) -> Scope2/1, Excitation System ST1A1/1(Upss)
  Mechanical DE/2(w) -> [f], PSS1/1(w), Governor/1(w)
  "Machine Equations "/2(Igxy1) -> pu->pu/1
  Vgxy/1 -> "Machine Equations "/2(Vgxy)
  "Machine Equations "/4(Vg) -> [Vg], Excitation System ST1A1/3(Vg)
  "Machine Equations "/1(Pe) -> [Pe], Mechanical DE/1(Pe), Scope1/1
  Excitation System ST1A1/1(Ef) -> "Machine Equations "/3(Ef), Scope5/1

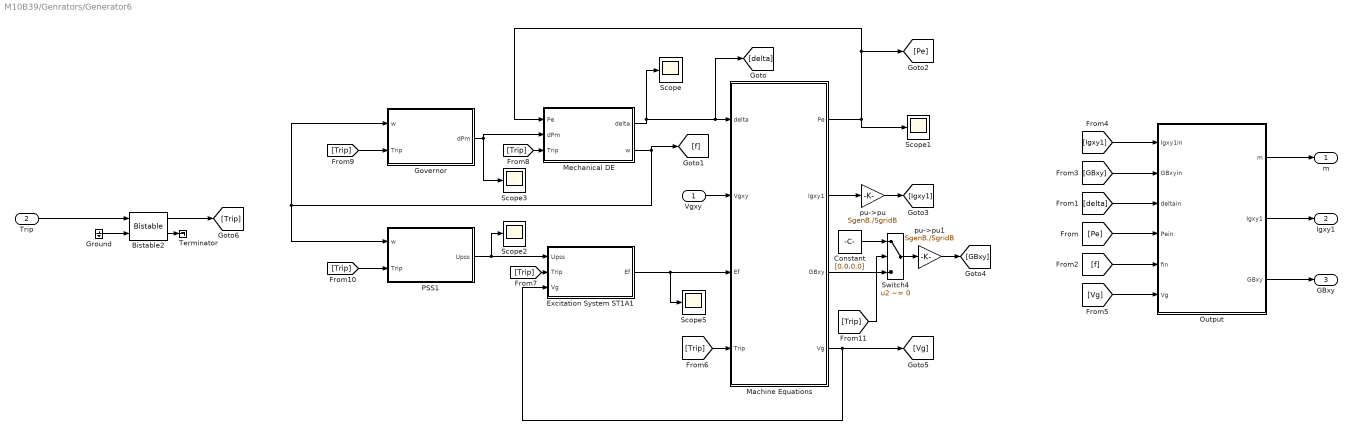
== system M10B39/Genrators/Generator6 ==
  Vgxy : Inport
  Trip : Inport  Port=2
  Bistable2 : powerlib_meascontrol/Logic/Bistable  Qpriority=Set  ic=0  Ts=0
  Constant : Constant  Value=[0,0,0,0]
  Excitation System ST1A1 : Subsystem
  Governor : Subsystem
  Ground : Ground
  "Machine Equations " : Subsystem
  Mechanical DE : Subsystem
  Output : Subsystem
  PSS1 : Subsystem
  Scope{,1..3,5} (5 alike) : Scope
  Switch4 : Switch  Criteria=u2 ~= 0  Threshold=0.5  SaturateOnIntegerOverflow=on
  Terminator : Terminator
  pu->pu : Gain  Gain=SgenB./SgridB
  pu->pu1 : Gain  Gain=SgenB./SgridB
  m : Outport
  Igxy1 : Outport  Port=2
  GBxy : Outport  Port=3
  wires:
  pu->pu1/1 -> [GBxy]
  pu->pu/1 -> [Igxy1]
  "Machine Equations "/3(GBxy) -> Switch4/3
  Constant/1 -> Switch4/1
  Switch4/1 -> pu->pu1/1
  [Trip] -> Switch4/2
  [Trip] -> PSS1/2(Trip)
  [Trip] -> Governor/2(Trip)
  [Trip] -> Mechanical DE/3(Trip)
  [Trip] -> Excitation System ST1A1/2(Trip)
  [Trip] -> "Machine Equations "/4(Trip)
  Bistable2/2 -> Terminator/1
  Trip/1 -> Bistable2/1
  Ground/1 -> Bistable2/2
  Bistable2/1 -> [Trip]
  [Vg] -> Output/6(Vg)
  Output/1(m) -> m/1
  Output/3(GBxy) -> GBxy/1
  Output/2(Igxy1) -> Igxy1/1
  [Igxy1] -> Output/1(Igxy1in)
  [GBxy] -> Output/2(GBxyin)
  [delta] -> Output/3(deltain)
  [f] -> Output/5(fin)
  [Pe] -> Output/4(Pein)
  Mechanical DE/1(delta) -> "Machine Equations "/1(delta), [delta], Scope/1
  Governor/1(dPm) -> Scope3/1, Mechanical DE/2(dPm)
  PSS1/1(Upss) -> Scope2/1, Excitation System ST1A1/1(Upss)
  Mechanical DE/2(w) -> [f], PSS1/1(w), Governor/1(w)
  "Machine Equations "/2(Igxy1) -> pu->pu/1
  Vgxy/1 -> "Machine Equations "/2(Vgxy)
  "Machine Equations "/4(Vg) -> [Vg], Excitation System ST1A1/3(Vg)
  "Machine Equations "/1(Pe) -> [Pe], Mechanical DE/1(Pe), Scope1/1
  Excitation System ST1A1/1(Ef) -> "Machine Equations "/3(Ef), Scope5/1

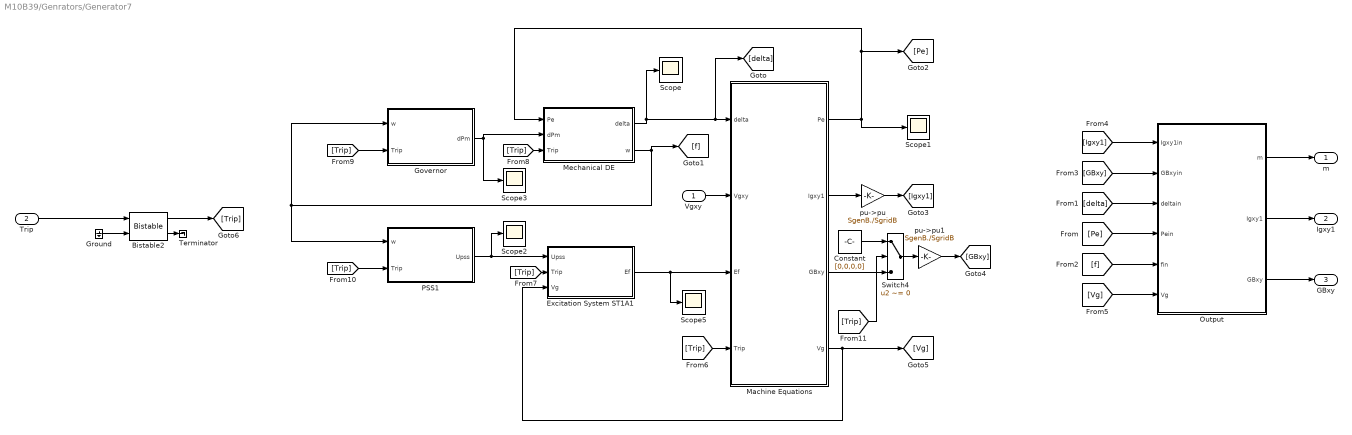
== system M10B39/Genrators/Generator7 ==
  Vgxy : Inport
  Trip : Inport  Port=2
  Bistable2 : powerlib_meascontrol/Logic/Bistable  Qpriority=Set  ic=0  Ts=0
  Constant : Constant  Value=[0,0,0,0]
  Excitation System ST1A1 : Subsystem
  Governor : Subsystem
  Ground : Ground
  "Machine Equations " : Subsystem
  Mechanical DE : Subsystem
  Output : Subsystem
  PSS1 : Subsystem
  Scope{,1..3,5} (5 alike) : Scope
  Switch4 : Switch  Criteria=u2 ~= 0  Threshold=0.5  SaturateOnIntegerOverflow=on
  Terminator : Terminator
  pu->pu : Gain  Gain=SgenB./SgridB
  pu->pu1 : Gain  Gain=SgenB./SgridB
  m : Outport
  Igxy1 : Outport  Port=2
  GBxy : Outport  Port=3
  wires:
  pu->pu1/1 -> [GBxy]
  pu->pu/1 -> [Igxy1]
  "Machine Equations "/3(GBxy) -> Switch4/3
  Constant/1 -> Switch4/1
  Switch4/1 -> pu->pu1/1
  [Trip] -> Switch4/2
  [Trip] -> PSS1/2(Trip)
  [Trip] -> Governor/2(Trip)
  [Trip] -> Mechanical DE/3(Trip)
  [Trip] -> Excitation System ST1A1/2(Trip)
  [Trip] -> "Machine Equations "/4(Trip)
  Bistable2/2 -> Terminator/1
  Trip/1 -> Bistable2/1
  Ground/1 -> Bistable2/2
  Bistable2/1 -> [Trip]
  [Vg] -> Output/6(Vg)
  Output/1(m) -> m/1
  Output/3(GBxy) -> GBxy/1
  Output/2(Igxy1) -> Igxy1/1
  [Igxy1] -> Output/1(Igxy1in)
  [GBxy] -> Output/2(GBxyin)
  [delta] -> Output/3(deltain)
  [f] -> Output/5(fin)
  [Pe] -> Output/4(Pein)
  Mechanical DE/1(delta) -> "Machine Equations "/1(delta), [delta], Scope/1
  Governor/1(dPm) -> Scope3/1, Mechanical DE/2(dPm)
  PSS1/1(Upss) -> Scope2/1, Excitation System ST1A1/1(Upss)
  Mechanical DE/2(w) -> [f], PSS1/1(w), Governor/1(w)
  "Machine Equations "/2(Igxy1) -> pu->pu/1
  Vgxy/1 -> "Machine Equations "/2(Vgxy)
  "Machine Equations "/4(Vg) -> [Vg], Excitation System ST1A1/3(Vg)
  "Machine Equations "/1(Pe) -> [Pe], Mechanical DE/1(Pe), Scope1/1
  Excitation System ST1A1/1(Ef) -> "Machine Equations "/3(Ef), Scope5/1

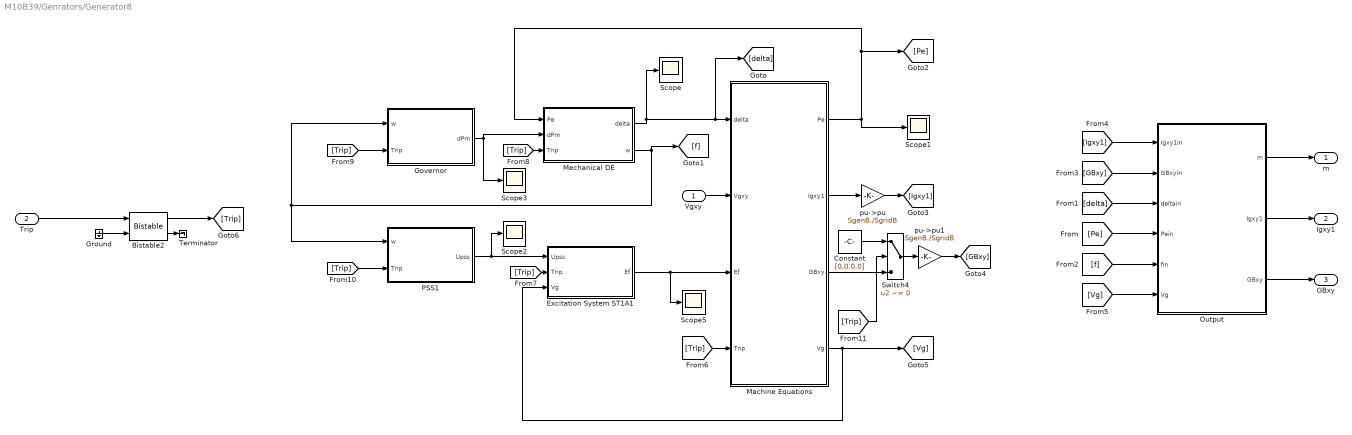
== system M10B39/Genrators/Generator8 ==
  Vgxy : Inport
  Trip : Inport  Port=2
  Bistable2 : powerlib_meascontrol/Logic/Bistable  Qpriority=Set  ic=0  Ts=0
  Constant : Constant  Value=[0,0,0,0]
  Excitation System ST1A1 : Subsystem
  Governor : Subsystem
  Ground : Ground
  "Machine Equations " : Subsystem
  Mechanical DE : Subsystem
  Output : Subsystem
  PSS1 : Subsystem
  Scope{,1..3,5} (5 alike) : Scope
  Switch4 : Switch  Criteria=u2 ~= 0  Threshold=0.5  SaturateOnIntegerOverflow=on
  Terminator : Terminator
  pu->pu : Gain  Gain=SgenB./SgridB
  pu->pu1 : Gain  Gain=SgenB./SgridB
  m : Outport
  Igxy1 : Outport  Port=2
  GBxy : Outport  Port=3
  wires:
  pu->pu1/1 -> [GBxy]
  pu->pu/1 -> [Igxy1]
  "Machine Equations "/3(GBxy) -> Switch4/3
  Constant/1 -> Switch4/1
  Switch4/1 -> pu->pu1/1
  [Trip] -> Switch4/2
  [Trip] -> PSS1/2(Trip)
  [Trip] -> Governor/2(Trip)
  [Trip] -> Mechanical DE/3(Trip)
  [Trip] -> Excitation System ST1A1/2(Trip)
  [Trip] -> "Machine Equations "/4(Trip)
  Bistable2/2 -> Terminator/1
  Trip/1 -> Bistable2/1
  Ground/1 -> Bistable2/2
  Bistable2/1 -> [Trip]
  [Vg] -> Output/6(Vg)
  Output/1(m) -> m/1
  Output/3(GBxy) -> GBxy/1
  Output/2(Igxy1) -> Igxy1/1
  [Igxy1] -> Output/1(Igxy1in)
  [GBxy] -> Output/2(GBxyin)
  [delta] -> Output/3(deltain)
  [f] -> Output/5(fin)
  [Pe] -> Output/4(Pein)
  Mechanical DE/1(delta) -> "Machine Equations "/1(delta), [delta], Scope/1
  Governor/1(dPm) -> Scope3/1, Mechanical DE/2(dPm)
  PSS1/1(Upss) -> Scope2/1, Excitation System ST1A1/1(Upss)
  Mechanical DE/2(w) -> [f], PSS1/1(w), Governor/1(w)
  "Machine Equations "/2(Igxy1) -> pu->pu/1
  Vgxy/1 -> "Machine Equations "/2(Vgxy)
  "Machine Equations "/4(Vg) -> [Vg], Excitation System ST1A1/3(Vg)
  "Machine Equations "/1(Pe) -> [Pe], Mechanical DE/1(Pe), Scope1/1
  Excitation System ST1A1/1(Ef) -> "Machine Equations "/3(Ef), Scope5/1

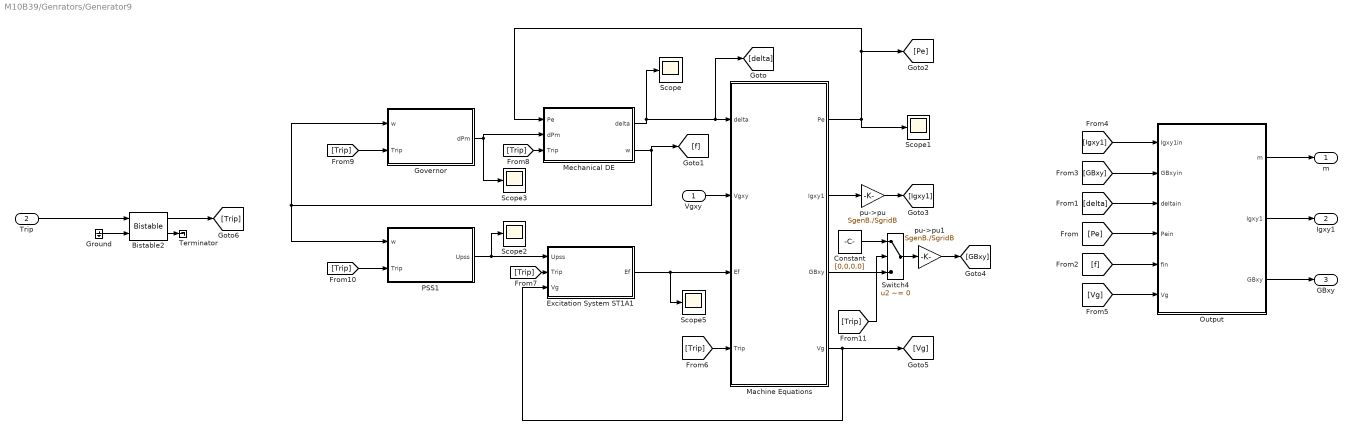
== system M10B39/Genrators/Generator9 ==
  Vgxy : Inport
  Trip : Inport  Port=2
  Bistable2 : powerlib_meascontrol/Logic/Bistable  Qpriority=Set  ic=0  Ts=0
  Constant : Constant  Value=[0,0,0,0]
  Excitation System ST1A1 : Subsystem
  Governor : Subsystem
  Ground : Ground
  "Machine Equations " : Subsystem
  Mechanical DE : Subsystem
  Output : Subsystem
  PSS1 : Subsystem
  Scope{,1..3,5} (5 alike) : Scope
  Switch4 : Switch  Criteria=u2 ~= 0  Threshold=0.5  SaturateOnIntegerOverflow=on
  Terminator : Terminator
  pu->pu : Gain  Gain=SgenB./SgridB
  pu->pu1 : Gain  Gain=SgenB./SgridB
  m : Outport
  Igxy1 : Outport  Port=2
  GBxy : Outport  Port=3
  wires:
  pu->pu1/1 -> [GBxy]
  pu->pu/1 -> [Igxy1]
  "Machine Equations "/3(GBxy) -> Switch4/3
  Constant/1 -> Switch4/1
  Switch4/1 -> pu->pu1/1
  [Trip] -> Switch4/2
  [Trip] -> PSS1/2(Trip)
  [Trip] -> Governor/2(Trip)
  [Trip] -> Mechanical DE/3(Trip)
  [Trip] -> Excitation System ST1A1/2(Trip)
  [Trip] -> "Machine Equations "/4(Trip)
  Bistable2/2 -> Terminator/1
  Trip/1 -> Bistable2/1
  Ground/1 -> Bistable2/2
  Bistable2/1 -> [Trip]
  [Vg] -> Output/6(Vg)
  Output/1(m) -> m/1
  Output/3(GBxy) -> GBxy/1
  Output/2(Igxy1) -> Igxy1/1
  [Igxy1] -> Output/1(Igxy1in)
  [GBxy] -> Output/2(GBxyin)
  [delta] -> Output/3(deltain)
  [f] -> Output/5(fin)
  [Pe] -> Output/4(Pein)
  Mechanical DE/1(delta) -> "Machine Equations "/1(delta), [delta], Scope/1
  Governor/1(dPm) -> Scope3/1, Mechanical DE/2(dPm)
  PSS1/1(Upss) -> Scope2/1, Excitation System ST1A1/1(Upss)
  Mechanical DE/2(w) -> [f], PSS1/1(w), Governor/1(w)
  "Machine Equations "/2(Igxy1) -> pu->pu/1
  Vgxy/1 -> "Machine Equations "/2(Vgxy)
  "Machine Equations "/4(Vg) -> [Vg], Excitation System ST1A1/3(Vg)
  "Machine Equations "/1(Pe) -> [Pe], Mechanical DE/1(Pe), Scope1/1
  Excitation System ST1A1/1(Ef) -> "Machine Equations "/3(Ef), Scope5/1

== system M10B39/Genrators/Generator1/Excitation System ST1A1 ==
  note: Ef
  Upss : Inport
  Trip : Inport  Port=2
  Vg : Inport  Port=3
  Constant1 : Constant  Value=0
  Ef1 : Integrator  InitialCondition=Ef10
  K : Gain  Gain=1/Tb  SaturateOnIntegerOverflow=on  OutDataTypeStr=Inherit: Same as input  ParamDataTypeStr=Inherit: Same as input
  KA : Gain  Gain=Ka  SaturateOnIntegerOverflow=on  OutDataTypeStr=Inherit: Same as input  ParamDataTypeStr=Inherit: Same as input
  KA1 : Gain  Gain=Tc/Tb  SaturateOnIntegerOverflow=on  OutDataTypeStr=Inherit: Same as input  ParamDataTypeStr=Inherit: Same as input
  KA2 : Gain  Gain=(1/Tb)*(1-Tc/Tb)  SaturateOnIntegerOverflow=on  OutDataTypeStr=Inherit: Same as input  ParamDataTypeStr=Inherit: Same as input
  Saturation : Saturate  UpperLimit=Efmax  LowerLimit=Efmin
  Sum : Sum  Inputs=|++  SaturateOnIntegerOverflow=on
  Sum1 : Sum  Inputs=|+-  SaturateOnIntegerOverflow=on
  Sum4 : Sum  Inputs=|+-+  SaturateOnIntegerOverflow=on
  Switch2 : Switch  Criteria=u2 ~= 0  Threshold=0.5  SaturateOnIntegerOverflow=on
  Switch3 : Switch  Criteria=u2 ~= 0  Threshold=0.5  SaturateOnIntegerOverflow=on
  Vref : Constant  Value=Vref
  Ef : Outport
  wires:
  Trip/1 -> Switch3/2, Switch2/2
  Constant1/1 -> Switch3/1, Switch2/1
  Switch3/1 -> KA2/1, K/1
  Ef1/1 -> Switch3/3
  Switch2/1 -> Ef1/1
  Sum1/1 -> Switch2/3
  KA/1 -> KA1/1, Sum1/1
  Upss/1 -> Sum4/3
  Saturation/1 -> Ef/1
  Vg/1 -> Sum4/2
  Sum4/1 -> KA/1
  Vref/1 -> Sum4/1
  Sum/1 -> Saturation/1
  K/1 -> Sum1/2
  KA1/1 -> Sum/2
  KA2/1 -> Sum/1

== system M10B39/Genrators/Generator1/Governor ==
  w : Inport
  Trip : Inport  Port=2
  CT : Constant  Value=0
  Constant : Constant  Value=0
  Gain : Gain  Gain=a_G  SaturateOnIntegerOverflow=on  OutDataTypeStr=Inherit: Same as input  ParamDataTypeStr=Inherit: Same as input
  Saturation : Saturate  UpperLimit=dPmax  LowerLimit=dPmin
  Sum1 : Sum  Inputs=|++  SaturateOnIntegerOverflow=on
  Sum3 : Sum  Inputs=|+-  SaturateOnIntegerOverflow=on
  Switch : Switch  Threshold=0.5  SaturateOnIntegerOverflow=on
  Switch1 : Switch  Criteria=u2 ~= 0  Threshold=0.5  SaturateOnIntegerOverflow=on
  Transfer Fcn1 : TransferFcn  Numerator=[b_G]  Denominator=[Tg_G 1]
  w0 : Gain  Gain=wB  SaturateOnIntegerOverflow=on  OutDataTypeStr=Inherit: Same as input  ParamDataTypeStr=Inherit: Same as input
  w1 : Constant  Value=S_Gov
  wref : Constant
  dPm : Outport
  wires:
  Gain/1 -> Sum1/1
  w1/1 -> Switch/2
  CT/1 -> Switch/3
  Sum3/1 -> w0/1
  Sum1/1 -> Saturation/1
  Saturation/1 -> Switch/1
  wref/1 -> Sum3/1
  w0/1 -> Gain/1, Transfer Fcn1/1
  Transfer Fcn1/1 -> Sum1/2
  w/1 -> Sum3/2
  Constant/1 -> Switch1/1
  Switch/1 -> Switch1/3
  Trip/1 -> Switch1/2
  Switch1/1 -> dPm/1

== system M10B39/Genrators/Generator1/Machine Equations  ==
  note: Iqg
  note: Idg
  note: 接口
  delta : Inport
  Vgxy : Inport  Port=2
  Ef : Inport  Port=3
  Trip : Inport  Port=4
  Demux : Demux  Outputs=2
  Demux1 : Demux  Outputs=2
  Fcn1 : Fcn  Expr=u(1)*u(3)+u(2)*u(4)
  Fcn2 : Fcn  Expr=(u(3)-u(2))/Xd1
  Fcn3 : Fcn  Expr=(u(1)-u(4))/Xq1
  Fcn4 : Fcn  Expr=u(2)*u(3)-u(1)*u(4)
  Fcn6 : Fcn  Expr=sqrt(u(1)^2+u(2)^2)
  Interface : Subsystem
  Mux1 : Mux  Inputs=2
  Mux2 : Mux  Inputs=2
  Mux3 : Mux  Inputs=2
  Qe : Scope
  Scope{,1..3} (4 alike) : Scope
  Transient Equations : Subsystem
  Pe : Outport
  Igxy1 : Outport  Port=2
  GBxy : Outport  Port=3
  Vg : Outport  Port=4
  wires:
  Trip/1 -> Transient Equations/3(Trip)
  Demux1/2 -> Scope3/1
  Demux/2 -> Scope2/1
  Demux1/1 -> Scope/1
  Demux/1 -> Scope1/1
  Transient Equations/1(Eqd') -> Interface/3(Eqd''), Mux1/2
  Interface/3(GBxy) -> GBxy/1
  Interface/2(Igxy1) -> Igxy1/1
  Vgxy/1 -> Interface/2(Vgxy)
  delta/1 -> Interface/1(delta)
  Fcn4/1 -> Qe/1
  Fcn6/1 -> Vg/1
  Fcn1/1 -> Pe/1
  Ef/1 -> Transient Equations/2(Ef)
  Mux2/1 -> Fcn4/1, Fcn1/1
  Mux1/1 -> Fcn3/1, Fcn2/1
  Interface/1(Vdqg) -> Mux1/1, Fcn6/1, Mux2/1, Demux/1
  Mux3/1 -> Mux2/2, Demux1/1, Transient Equations/1(Idqg)
  Fcn2/1 -> Mux3/1
  Fcn3/1 -> Mux3/2

== system M10B39/Genrators/Generator1/Mechanical DE ==
  Pe : Inport
  dPm : Inport  Port=2
  Trip : Inport  Port=3
  Constant1 : Constant  Value=0
  Constant2 : Constant  Value=0
  Gain : Gain  Gain=wB  SaturateOnIntegerOverflow=on  OutDataTypeStr=Inherit: Same as input  ParamDataTypeStr=Inherit: Same as input
  Gain1 : Gain  Gain=1/H  SaturateOnIntegerOverflow=on  OutDataTypeStr=Inherit: Same as input  ParamDataTypeStr=Inherit: Same as input
  Gain2 : Gain  Gain=D  SaturateOnIntegerOverflow=on  OutDataTypeStr=Inherit: Same as input  ParamDataTypeStr=Inherit: Same as input
  Gain5 : Gain  Gain=180/pi  SaturateOnIntegerOverflow=on  OutDataTypeStr=Inherit: Same as input  ParamDataTypeStr=Inherit: Same as input
  Int1 : Integrator  InitialCondition=delta0
  Int2 : Integrator  InitialCondition=w0
  Pm : Constant  Value=Pm0
  Scope2 : Scope
  Scope4 : Scope
  Scope8 : Scope
  Sum2 : Sum  Inputs=-+-+  SaturateOnIntegerOverflow=on
  Sum3 : Sum  Inputs=|+-  SaturateOnIntegerOverflow=on
  Switch{1..4} (4 alike) : Switch  Criteria=u2 ~= 0  Threshold=0.5  SaturateOnIntegerOverflow=on
  w0 : Constant
  delta : Outport
  w : Outport  Port=2
  wires:
  [Trip] -> Switch3/2, Switch2/2
  Constant1/1 -> Switch3/1, Switch2/1
  Switch3/1 -> Scope4/1, Sum3/1, w/1
  Int2/1 -> Switch3/3
  Switch2/1 -> Int2/1
  Gain1/1 -> Switch2/3
  Trip/1 -> [Trip]
  [Trip] -> Switch1/2, Switch4/2
  Constant2/1 -> Switch4/1, Switch1/1
  Switch4/1 -> delta/1, Scope2/1, Gain5/1
  Int1/1 -> Switch4/3
  Switch1/1 -> Int1/1
  Gain/1 -> Switch1/3
  Gain5/1 -> Scope8/1
  w0/1 -> Sum3/2
  Sum3/1 -> Gain2/1, Gain/1
  Pm/1 -> Sum2/2
  Gain2/1 -> Sum2/1
  Sum2/1 -> Gain1/1
  Pe/1 -> Sum2/3
  dPm/1 -> Sum2/4

== system M10B39/Genrators/Generator1/Output ==
  Igxy1in : Inport
  GBxyin : Inport  Port=2
  deltain : Inport  Port=3
  Pein : Inport  Port=4
  fin : Inport  Port=5
  Vg : Inport  Port=6
  Bus Creator : BusCreator  Inputs=6
  m : Outport
  Igxy1 : Outport  Port=2
  GBxy : Outport  Port=3
  wires:
  Vg/1 -> Bus Creator/6  "Vg"
  fin/1 -> Bus Creator/5  "f"
  Pein/1 -> Bus Creator/4  "Pe"
  deltain/1 -> Bus Creator/3  "delta"
  GBxyin/1 -> Bus Creator/2, GBxy/1  "GBxy"
  Igxy1in/1 -> Bus Creator/1, Igxy1/1  "Igxy1"
  Bus Creator/1 -> m/1

== system M10B39/Genrators/Generator1/PSS1 ==
  w : Inport
  Trip : Inport  Port=2
  CT : Constant  Value=0
  Constant : Constant  Value=0
  Gain : Gain  Gain=Kpss  SaturateOnIntegerOverflow=on  OutDataTypeStr=Inherit: Same as input  ParamDataTypeStr=Inherit: Same as input
  Saturation : Saturate  UpperLimit=Upmax  LowerLimit=Upmin
  Sum3 : Sum  Inputs=|+-  SaturateOnIntegerOverflow=on
  Switch : Switch  Threshold=0.5  SaturateOnIntegerOverflow=on
  Switch1 : Switch  Threshold=0.5  SaturateOnIntegerOverflow=on
  Transfer Fcn : TransferFcn  Numerator=[Tw_P 0]  Denominator=[Tw_P 1]
  Transfer Fcn1 : TransferFcn  Numerator=[T1_P 1]  Denominator=[T2_P 1]
  Transfer Fcn2 : TransferFcn  Numerator=[T3_P 1]  Denominator=[T4_P 1]
  w0 : Constant
  w1 : Constant  Value=S_PSS
  Upss : Outport
  wires:
  Constant/1 -> Switch1/1
  Trip/1 -> Switch1/2
  Switch1/1 -> Upss/1
  Switch/1 -> Switch1/3
  Transfer Fcn/1 -> Transfer Fcn1/1
  Gain/1 -> Transfer Fcn/1
  w1/1 -> Switch/2
  CT/1 -> Switch/3
  Saturation/1 -> Switch/1
  Sum3/1 -> Gain/1
  Transfer Fcn2/1 -> Saturation/1
  Transfer Fcn1/1 -> Transfer Fcn2/1
  w/1 -> Sum3/1
  w0/1 -> Sum3/2

== system M10B39/Genrators/Generator10/Excitation System ST1A1 ==
  note: Ef
  Upss : Inport
  Trip : Inport  Port=2
  Vg : Inport  Port=3
  Constant1 : Constant  Value=0
  Ef1 : Integrator  InitialCondition=Ef10
  K : Gain  Gain=1/Tb  SaturateOnIntegerOverflow=on  OutDataTypeStr=Inherit: Same as input  ParamDataTypeStr=Inherit: Same as input
  KA : Gain  Gain=Ka  SaturateOnIntegerOverflow=on  OutDataTypeStr=Inherit: Same as input  ParamDataTypeStr=Inherit: Same as input
  KA1 : Gain  Gain=Tc/Tb  SaturateOnIntegerOverflow=on  OutDataTypeStr=Inherit: Same as input  ParamDataTypeStr=Inherit: Same as input
  KA2 : Gain  Gain=(1/Tb)*(1-Tc/Tb)  SaturateOnIntegerOverflow=on  OutDataTypeStr=Inherit: Same as input  ParamDataTypeStr=Inherit: Same as input
  Saturation : Saturate  UpperLimit=Efmax  LowerLimit=Efmin
  Sum : Sum  Inputs=|++  SaturateOnIntegerOverflow=on
  Sum1 : Sum  Inputs=|+-  SaturateOnIntegerOverflow=on
  Sum4 : Sum  Inputs=|+-+  SaturateOnIntegerOverflow=on
  Switch2 : Switch  Criteria=u2 ~= 0  Threshold=0.5  SaturateOnIntegerOverflow=on
  Switch3 : Switch  Criteria=u2 ~= 0  Threshold=0.5  SaturateOnIntegerOverflow=on
  Vref : Constant  Value=Vref
  Ef : Outport
  wires:
  Trip/1 -> Switch3/2, Switch2/2
  Constant1/1 -> Switch3/1, Switch2/1
  Switch3/1 -> KA2/1, K/1
  Ef1/1 -> Switch3/3
  Switch2/1 -> Ef1/1
  Sum1/1 -> Switch2/3
  KA/1 -> KA1/1, Sum1/1
  Upss/1 -> Sum4/3
  Saturation/1 -> Ef/1
  Vg/1 -> Sum4/2
  Sum4/1 -> KA/1
  Vref/1 -> Sum4/1
  Sum/1 -> Saturation/1
  K/1 -> Sum1/2
  KA1/1 -> Sum/2
  KA2/1 -> Sum/1

== system M10B39/Genrators/Generator10/Governor ==
  w : Inport
  Trip : Inport  Port=2
  CT : Constant  Value=0
  Constant : Constant  Value=0
  Gain : Gain  Gain=a_G  SaturateOnIntegerOverflow=on  OutDataTypeStr=Inherit: Same as input  ParamDataTypeStr=Inherit: Same as input
  Saturation : Saturate  UpperLimit=dPmax  LowerLimit=dPmin
  Sum1 : Sum  Inputs=|++  SaturateOnIntegerOverflow=on
  Sum3 : Sum  Inputs=|+-  SaturateOnIntegerOverflow=on
  Switch : Switch  Threshold=0.5  SaturateOnIntegerOverflow=on
  Switch1 : Switch  Criteria=u2 ~= 0  Threshold=0.5  SaturateOnIntegerOverflow=on
  Transfer Fcn1 : TransferFcn  Numerator=[b_G]  Denominator=[Tg_G 1]
  w0 : Gain  Gain=wB  SaturateOnIntegerOverflow=on  OutDataTypeStr=Inherit: Same as input  ParamDataTypeStr=Inherit: Same as input
  w1 : Constant  Value=S_Gov
  wref : Constant
  dPm : Outport
  wires:
  Gain/1 -> Sum1/1
  w1/1 -> Switch/2
  CT/1 -> Switch/3
  Sum3/1 -> w0/1
  Sum1/1 -> Saturation/1
  Saturation/1 -> Switch/1
  wref/1 -> Sum3/1
  w0/1 -> Gain/1, Transfer Fcn1/1
  Transfer Fcn1/1 -> Sum1/2
  w/1 -> Sum3/2
  Constant/1 -> Switch1/1
  Switch/1 -> Switch1/3
  Trip/1 -> Switch1/2
  Switch1/1 -> dPm/1

== system M10B39/Genrators/Generator10/Machine Equations  ==
  note: Iqg
  note: Idg
  note: 接口
  delta : Inport
  Vgxy : Inport  Port=2
  Ef : Inport  Port=3
  Trip : Inport  Port=4
  Demux : Demux  Outputs=2
  Demux1 : Demux  Outputs=2
  Fcn1 : Fcn  Expr=u(1)*u(3)+u(2)*u(4)
  Fcn2 : Fcn  Expr=(u(3)-u(2))/Xd1
  Fcn3 : Fcn  Expr=(u(1)-u(4))/Xq1
  Fcn4 : Fcn  Expr=u(2)*u(3)-u(1)*u(4)
  Fcn6 : Fcn  Expr=sqrt(u(1)^2+u(2)^2)
  Interface : Subsystem
  Mux1 : Mux  Inputs=2
  Mux2 : Mux  Inputs=2
  Mux3 : Mux  Inputs=2
  Qe : Scope
  Scope{,1..3} (4 alike) : Scope
  Transient Equations : Subsystem
  Pe : Outport
  Igxy1 : Outport  Port=2
  GBxy : Outport  Port=3
  Vg : Outport  Port=4
  wires:
  Trip/1 -> Transient Equations/3(Trip)
  Demux1/2 -> Scope3/1
  Demux/2 -> Scope2/1
  Demux1/1 -> Scope/1
  Demux/1 -> Scope1/1
  Transient Equations/1(Eqd') -> Interface/3(Eqd''), Mux1/2
  Interface/3(GBxy) -> GBxy/1
  Interface/2(Igxy1) -> Igxy1/1
  Vgxy/1 -> Interface/2(Vgxy)
  delta/1 -> Interface/1(delta)
  Fcn4/1 -> Qe/1
  Fcn6/1 -> Vg/1
  Fcn1/1 -> Pe/1
  Ef/1 -> Transient Equations/2(Ef)
  Mux2/1 -> Fcn4/1, Fcn1/1
  Mux1/1 -> Fcn3/1, Fcn2/1
  Interface/1(Vdqg) -> Mux1/1, Fcn6/1, Mux2/1, Demux/1
  Mux3/1 -> Mux2/2, Demux1/1, Transient Equations/1(Idqg)
  Fcn2/1 -> Mux3/1
  Fcn3/1 -> Mux3/2
